simulink model "VCMGCM1962020b_v2"  (R2020b)
settings: Solver=FixedStepDiscrete  StartTime=0.0  StopTime=10.0  FixedStep=0.005  RelTol=1e-3  EnableMultiTasking=on
PreLoadFcn:
  | try, model_open; catch, disp('Error occurred while executing model pre-load callback: model_open.m'); disp('Please assure that the MATLAB working directory is set to the model directory before opening.'); end
InitFcn:
  | try, model_open; catch, end
undefined symbols (not defined in the file): Bridge, GCM, H, raptor_get_param_eval, raptor_get_safe_string, raptor_xcp_function
libraries: Blocks_lib x1165, Raptor_lib x665, simulink x62, VCM_lib x5
(part 5 of 23)

== system VCMGCM1962020b_v2/Fgnd/Diagnostics/Fault Statuses/Status Marquees ==
  f : TriggerPort  TriggerType=function-call  VariantControl=(inherit)  PortDimensions=1
  Display first 7 faults with the selected state1 : Subsystem  mask{group=group, notOccurred=off, suspected=off, active=off, occurred=off, failedThisDC=off, testCmpltThisDC=off, failing=on, pending=off, confirmed=off, mil=off, permanent=off, ready=off, prevConfirmed=off, failedSinceClear=off, failedLastDC=off, prevMil=off}
      mask prompts: notOccurred "Not Occurred"; failedThisDC "Failed This Drive Cycle"; testCmpltThisDC "Test Completed This Drive Cycle"; prevConfirmed "Previously Confirmed"; failedSinceClear "Failed Since Last Clear"; failedLastDC "FailedLastDriveCycle"; prevMil "Previously MIL"
      mask init:
      | %names used in Raptor
      | %OBD1:
      | %maskVarList = {'notOccurred' ; 'suspected'; 'active'; 'occurred'};
      | %OBD2:
      | maskVarList = {'notOccurred' ; 'suspected'; 'active'; 'occurred'; 'failedThisDC'; 'testCmpltThisDC'; 'failing'; 'pending'; 'confirmed'; 'mil'; 'permanent'; 'ready'; 'prevConfirmed'; 'failedSinceClear'; 'failedLastDC'; 'prevMil'};
      | %cleaner names to use in actual variable names
      | %OBD1:
      | %outputNameList= {'NotOccurred'; 'Suspected'; 'Active'; 'Occurred'};
      | %OBD2:
      | outputNameList = {'notOccurred' ; 'suspected'; 'active'; 'occurred'; 'FailThisDrv' ; 'CmpltThisDrv'   ; 'Failing'; 'Pending'; 'Confirmed'; 'MIL'; 'Permanent'; 'Ready'; 'PrevConfirmed'; 'FaildSinceClr'   ; 'FaildLastDrv'; 'PrevMIL'};
      | 
      | debug = [];
      | isSelected = cell(0);
      | selectedOutputNames = [];
      | for i = 1:length(maskVarList)
      |     paramVal = eval(maskVarList{i});
      |     if paramVal %if that fault is selected
      |         selectedOutputNames = [selectedOutputNames outputNameList{i}];
      |         isSelected = [isSelected 'on'];
      |     else
      |         isSelected = [isSelected 'off'];
      |     end
      | end
      | 
      | finalVarName = selectedOutputNames; %concatenate all names
      | debug = finalVarName;
      | 
      | iterators = find_system(gcb,'LookUnderMasks','all','FunctionName','raptor_sfun_fault_stateIterator');
      | countBlk = find_system(gcb,'LookUnderMasks','all','FunctionName','raptor_sfun_fault_stateCount');
      | blocks = [iterators; countBlk]; %blocks that need to be configured
      | 
      | for b = 1:length(blocks)
      |     for v = 1:length(maskVarList)
      |         set_param(blocks{b},maskVarList{v},isSelected{v});
      |     end    
      | end
      mask Display: disp(finalVarName)
  Display first 7 faults with the selected state2 : Subsystem  mask{group=group, notOccurred=off, suspected=off, active=off, occurred=off, failedThisDC=on, testCmpltThisDC=off, failing=off, pending=off, confirmed=off, mil=off, permanent=off, ready=off, prevConfirmed=off, failedSinceClear=off, failedLastDC=off, prevMil=off}
      mask prompts: notOccurred "Not Occurred"; failedThisDC "Failed This Drive Cycle"; testCmpltThisDC "Test Completed This Drive Cycle"; prevConfirmed "Previously Confirmed"; failedSinceClear "Failed Since Last Clear"; failedLastDC "FailedLastDriveCycle"; prevMil "Previously MIL"
      mask init: same as VCMGCM1962020b_v2/Fgnd/Diagnostics/Fault Statuses/Status Marquees/Display first 7 faults with the selected state1
      mask Display: disp(finalVarName)
  Fault Fail Time : Subsystem  TreatAsAtomicUnit=on
  Header : Blocks_lib/Header  width=Portrait  addtext=''
  Unit Delay{,1..6} (7 alike) : UnitDelay  SampleTime=-1  HasFrameUpgradeWarning=on
  raptor_fault_data_read : Raptor_lib/Faults/raptor_fault_data_read  dataSource=Parameter  dataName='FaultFailTime'  faultSource=Port  faultName='myFaultName'
      settings: SourceProductName=Raptor
  raptor_fault_measurement : Raptor_lib/Faults/raptor_fault_measurement  dataName='TestCompletedThisDriveCycleFaults'  calHelp='Marquee of test completed this drive cycle faults'  calAccess=1  calFunction=group
      settings: SourceProductName=Raptor
  raptor_fault_measurement1 : Raptor_lib/Faults/raptor_fault_measurement  dataName='FailingFaults'  calHelp='Marquee of failing faults'  calAccess=1  calFunction=group
      settings: SourceProductName=Raptor
  raptor_fault_measurement2 : Raptor_lib/Faults/raptor_fault_measurement  dataName='FailedThisDriveCycleFaults'  calHelp='Marquee of failed this drive cycle faults'  calAccess=1  calFunction=group
      settings: SourceProductName=Raptor
  raptor_fault_measurement3 : Raptor_lib/Faults/raptor_fault_measurement  dataName='FailedSinceClearFaults'  calHelp='Marquee of failed since clear faults'  calAccess=1  calFunction=group
      settings: SourceProductName=Raptor
  raptor_fault_measurement4 : Raptor_lib/Faults/raptor_fault_measurement  dataName='PendingFaults'  calHelp='Marquee of pending faults'  calAccess=1  calFunction=group
      settings: SourceProductName=Raptor
  raptor_fault_measurement5 : Raptor_lib/Faults/raptor_fault_measurement  dataName='ConfirmedFaults'  calHelp='Marquee of confirmed faults'  calAccess=1  calFunction=group
      settings: SourceProductName=Raptor
  raptor_fault_measurement6 : Raptor_lib/Faults/raptor_fault_measurement  dataName='PreviouslyConfirmedFaults'  calHelp='Marquee of previously confirmed faults'  calAccess=1  calFunction=group
      settings: SourceProductName=Raptor
  raptor_fault_stateIterator : Raptor_lib/Faults/raptor_fault_stateIterator  notOccurred=off  suspected=off  active=on  occurred=off  failedThisDC=off  testCmpltThisDC=on  failing=off  pending=off  confirmed=off  mil=off  permanent=off  ready=off  prevConfirmed=off  failedSinceClear=off  failedLastDC=off  prevMil=off
      settings: SourceProductName=Raptor
  raptor_fault_stateIterator1 : Raptor_lib/Faults/raptor_fault_stateIterator  notOccurred=off  suspected=off  active=on  occurred=off  failedThisDC=off  testCmpltThisDC=off  failing=on  pending=off  confirmed=off  mil=off  permanent=off  ready=off  prevConfirmed=off  failedSinceClear=off  failedLastDC=off  prevMil=off
      settings: SourceProductName=Raptor
  raptor_fault_stateIterator2 : Raptor_lib/Faults/raptor_fault_stateIterator  notOccurred=off  suspected=off  active=on  occurred=off  failedThisDC=on  testCmpltThisDC=off  failing=off  pending=off  confirmed=off  mil=off  permanent=off  ready=off  prevConfirmed=off  failedSinceClear=off  failedLastDC=off  prevMil=off
      settings: SourceProductName=Raptor
  raptor_fault_stateIterator3 : Raptor_lib/Faults/raptor_fault_stateIterator  notOccurred=off  suspected=off  active=on  occurred=off  failedThisDC=off  testCmpltThisDC=off  failing=off  pending=off  confirmed=off  mil=off  permanent=off  ready=off  prevConfirmed=off  failedSinceClear=on  failedLastDC=off  prevMil=off
      settings: SourceProductName=Raptor
  raptor_fault_stateIterator4 : Raptor_lib/Faults/raptor_fault_stateIterator  notOccurred=off  suspected=off  active=on  occurred=off  failedThisDC=off  testCmpltThisDC=off  failing=off  pending=on  confirmed=off  mil=off  permanent=off  ready=off  prevConfirmed=off  failedSinceClear=off  failedLastDC=off  prevMil=off
      settings: SourceProductName=Raptor
  raptor_fault_stateIterator5 : Raptor_lib/Faults/raptor_fault_stateIterator  notOccurred=off  suspected=off  active=on  occurred=off  failedThisDC=off  testCmpltThisDC=off  failing=off  pending=off  confirmed=on  mil=off  permanent=off  ready=off  prevConfirmed=off  failedSinceClear=off  failedLastDC=off  prevMil=off
      settings: SourceProductName=Raptor
  raptor_fault_stateIterator6 : Raptor_lib/Faults/raptor_fault_stateIterator  notOccurred=off  suspected=off  active=on  occurred=off  failedThisDC=off  testCmpltThisDC=off  failing=off  pending=off  confirmed=off  mil=off  permanent=off  ready=off  prevConfirmed=on  failedSinceClear=off  failedLastDC=off  prevMil=off
      settings: SourceProductName=Raptor
  raptor_fault_trigger : Raptor_lib/Faults/raptor_fault_trigger  triggerName='FailingTime'  setGlobal=on  stdState=Suspected  obdState=Failing  edge=Rising  alwaysEnabled=on
      settings: SourceProductName=Raptor
  raptor_measurement : Raptor_lib/Data Storage/raptor_measurement  paramName='FailedThisDriveCycleFaultsTime'  nameSource=Parameter  calDispType=Number  calEnum={'False', 'True'}  calGain=1.0  calOffset=0.0  calMax=inf  calMin=-inf  calFormat='-1'  calUnit='Marquee of failed this drive cycle faults time'  calHelp='sec'  calAccess=1  calFunction=group  calVisible=on
      settings: SourceProductName=Raptor
  wires:
  raptor_fault_stateIterator/1 -> raptor_fault_measurement/1, Unit Delay/1
  Unit Delay/1 -> raptor_fault_stateIterator/1
  Unit Delay1/1 -> raptor_fault_stateIterator1/1
  raptor_fault_stateIterator1/1 -> Unit Delay1/1, raptor_fault_measurement1/1
  raptor_fault_stateIterator2/1 -> raptor_fault_measurement2/1, raptor_fault_data_read/1, Unit Delay2/1
  Unit Delay2/1 -> raptor_fault_stateIterator2/1
  Unit Delay3/1 -> raptor_fault_stateIterator3/1
  raptor_fault_stateIterator3/1 -> Unit Delay3/1, raptor_fault_measurement3/1
  raptor_fault_stateIterator4/1 -> raptor_fault_measurement4/1, Unit Delay4/1
  Unit Delay4/1 -> raptor_fault_stateIterator4/1
  Unit Delay5/1 -> raptor_fault_stateIterator5/1
  raptor_fault_stateIterator5/1 -> Unit Delay5/1, raptor_fault_measurement5/1
  raptor_fault_stateIterator6/1 -> raptor_fault_measurement6/1, Unit Delay6/1
  Unit Delay6/1 -> raptor_fault_stateIterator6/1
  raptor_fault_trigger/2 -> Fault Fail Time/1(Idx)
  raptor_fault_trigger/1 -> Fault Fail Time/Trigger
  raptor_fault_data_read/1 -> raptor_measurement/1

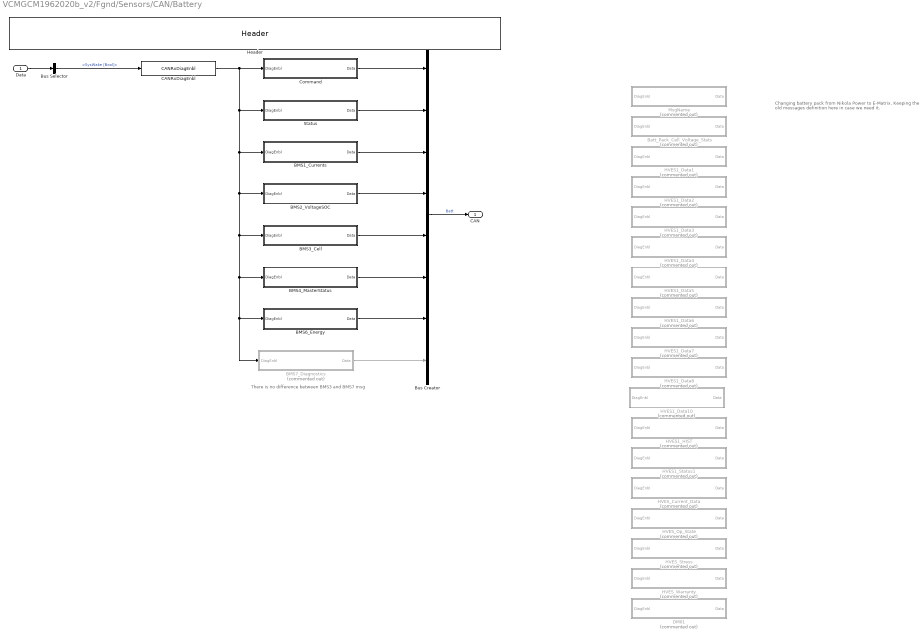
== system VCMGCM1962020b_v2/Fgnd/Sensors/CAN/Battery ==
  note: There is no difference between BMS3 and BMS7 msg
  note: Changing battery pack from Nikola Power to E-Matrix.
      | Keeping the old messages definition here in case we need it.
  Data : Inport
  BMS1_Currents : Subsystem  mask{samptime=samptime}
      mask prompts: samptime "Sample Time (sec)"
      mask help:
      | Example of how to set up a CAN message recieve.
      | 1. Copy this block into the main model.
      | 2. Disable/break library link.
      | 3. Underneath, set up CAN Rx Message block.
      | 4. For each field, connect a CANRxField block from the CAN block to the bus creator; adjust parameters as necessary.
      mask init:
      | [msgnam, msgbus] = CANBlockInit('Rx');
      mask Display: disp(['CAN Rx: Message\n' msgnam '\n' msgbus]);
  BMS2_VoltageSOC : Subsystem  AncestorBlock=Blocks_lib/MsgName5  mask{samptime=0.005}
      mask prompts: samptime "Sample Time (sec)"
      mask help:
      | Example of how to set up a CAN message recieve.
      | 1. Copy this block into the main model.
      | 2. Disable/break library link.
      | 3. Underneath, set up CAN Rx Message block.
      | 4. For each field, connect a CANRxField block from the CAN block to the bus creator; adjust parameters as necessary.
      mask init:
      | [msgnam, msgbus] = CANBlockInit('Rx');
      mask Display: disp(['CAN Rx: Message\n' msgnam '\n' msgbus]);
  BMS3_Cell : Subsystem  mask{samptime=samptime}
      mask prompts: samptime "Sample Time (sec)"
      mask help:
      | Example of how to set up a CAN message recieve.
      | 1. Copy this block into the main model.
      | 2. Disable/break library link.
      | 3. Underneath, set up CAN Rx Message block.
      | 4. For each field, connect a CANRxField block from the CAN block to the bus creator; adjust parameters as necessary.
      mask init:
      | [msgnam, msgbus] = CANBlockInit('Rx');
      mask Display: disp(['CAN Rx: Message\n' msgnam '\n' msgbus]);
  BMS4_MasterStatus : Subsystem  mask{samptime=samptime}
      mask prompts: samptime "Sample Time (sec)"
      mask help:
      | Example of how to set up a CAN message recieve.
      | 1. Copy this block into the main model.
      | 2. Disable/break library link.
      | 3. Underneath, set up CAN Rx Message block.
      | 4. For each field, connect a CANRxField block from the CAN block to the bus creator; adjust parameters as necessary.
      mask init:
      | [msgnam, msgbus] = CANBlockInit('Rx');
      mask Display: disp(['CAN Rx: Message\n' msgnam '\n' msgbus]);
  BMS6_Energy : Subsystem  mask{samptime=samptime}
      mask prompts: samptime "Sample Time (sec)"
      mask help:
      | Example of how to set up a CAN message recieve.
      | 1. Copy this block into the main model.
      | 2. Disable/break library link.
      | 3. Underneath, set up CAN Rx Message block.
      | 4. For each field, connect a CANRxField block from the CAN block to the bus creator; adjust parameters as necessary.
      mask init:
      | [msgnam, msgbus] = CANBlockInit('Rx');
      mask Display: disp(['CAN Rx: Message\n' msgnam '\n' msgbus]);
  BMS7_Diagnostics : Subsystem  Commented=on  mask{samptime=samptime}
      mask prompts: samptime "Sample Time (sec)"
      mask help:
      | Example of how to set up a CAN message recieve.
      | 1. Copy this block into the main model.
      | 2. Disable/break library link.
      | 3. Underneath, set up CAN Rx Message block.
      | 4. For each field, connect a CANRxField block from the CAN block to the bus creator; adjust parameters as necessary.
      mask init:
      | [msgnam, msgbus] = CANBlockInit('Rx');
      mask Display: disp(['CAN Rx: Message\n' msgnam '\n' msgbus]);
  Batt_Pack_Cell_Voltage_Stats : Subsystem  Commented=on  mask{samptime=samptime}
      mask prompts: samptime "Sample Time (sec)"
      mask help:
      | Example of how to set up a CAN message recieve.
      | 1. Copy this block into the main model.
      | 2. Disable/break library link.
      | 3. Underneath, set up CAN Rx Message block.
      | 4. For each field, connect a CANRxField block from the CAN block to the bus creator; adjust parameters as necessary.
      mask init:
      | [msgnam, msgbus] = CANBlockInit('Rx');
      mask Display: disp(['CAN Rx: Message\n' msgnam '\n' msgbus]);
  Bus Creator : BusCreator  Inputs=8
  Bus Selector : BusSelector  OutputSignals=Control.Other.Other.SysWake [Bool]
  CANRxDiagEnbl : Blocks_lib/CANRxDiagEnbl  nam='Batt'
  Command : Subsystem  mask{samptime=samptime}
      mask prompts: samptime "Sample Time (sec)"
      mask help:
      | Example of how to set up a CAN message recieve.
      | 1. Copy this block into the main model.
      | 2. Disable/break library link.
      | 3. Underneath, set up CAN Rx Message block.
      | 4. For each field, connect a CANRxField block from the CAN block to the bus creator; adjust parameters as necessary.
      mask init:
      | [msgnam, msgbus] = CANBlockInit('Rx');
      mask Display: disp(['CAN Rx: Message\n' msgnam '\n' msgbus]);
  DM01 : Subsystem  Commented=on  mask{samptime=samptime}
      mask prompts: samptime "Sample Time (sec)"
      mask help:
      | Example of how to set up a CAN message recieve.
      | 1. Copy this block into the main model.
      | 2. Disable/break library link.
      | 3. Underneath, set up CAN Rx Message block.
      | 4. For each field, connect a CANRxField block from the CAN block to the bus creator; adjust parameters as necessary.
      mask init:
      | [msgnam, msgbus] = CANBlockInit('Rx');
      mask Display: disp(['CAN Rx: Message\n' msgnam '\n' msgbus]);
  HVES1_Data1 : Subsystem  Commented=on  mask{samptime=samptime}
      mask prompts: samptime "Sample Time (sec)"
      mask help:
      | Example of how to set up a CAN message recieve.
      | 1. Copy this block into the main model.
      | 2. Disable/break library link.
      | 3. Underneath, set up CAN Rx Message block.
      | 4. For each field, connect a CANRxField block from the CAN block to the bus creator; adjust parameters as necessary.
      mask init:
      | [msgnam, msgbus] = CANBlockInit('Rx');
      mask Display: disp(['CAN Rx: Message\n' msgnam '\n' msgbus]);
  HVES1_Data10 : Subsystem  Commented=on  mask{samptime=samptime}
      mask prompts: samptime "Sample Time (sec)"
      mask help:
      | Example of how to set up a CAN message recieve.
      | 1. Copy this block into the main model.
      | 2. Disable/break library link.
      | 3. Underneath, set up CAN Rx Message block.
      | 4. For each field, connect a CANRxField block from the CAN block to the bus creator; adjust parameters as necessary.
      mask init:
      | [msgnam, msgbus] = CANBlockInit('Rx');
      mask Display: disp(['CAN Rx: Message\n' msgnam '\n' msgbus]);
  HVES1_Data2 : Subsystem  Commented=on  mask{samptime=samptime}
      mask prompts: samptime "Sample Time (sec)"
      mask help:
      | Example of how to set up a CAN message recieve.
      | 1. Copy this block into the main model.
      | 2. Disable/break library link.
      | 3. Underneath, set up CAN Rx Message block.
      | 4. For each field, connect a CANRxField block from the CAN block to the bus creator; adjust parameters as necessary.
      mask init:
      | [msgnam, msgbus] = CANBlockInit('Rx');
      mask Display: disp(['CAN Rx: Message\n' msgnam '\n' msgbus]);
  HVES1_Data3 : Subsystem  Commented=on  mask{samptime=samptime}
      mask prompts: samptime "Sample Time (sec)"
      mask help:
      | Example of how to set up a CAN message recieve.
      | 1. Copy this block into the main model.
      | 2. Disable/break library link.
      | 3. Underneath, set up CAN Rx Message block.
      | 4. For each field, connect a CANRxField block from the CAN block to the bus creator; adjust parameters as necessary.
      mask init:
      | [msgnam, msgbus] = CANBlockInit('Rx');
      mask Display: disp(['CAN Rx: Message\n' msgnam '\n' msgbus]);
  HVES1_Data4 : Subsystem  Commented=on  mask{samptime=samptime}
      mask prompts: samptime "Sample Time (sec)"
      mask help:
      | Example of how to set up a CAN message recieve.
      | 1. Copy this block into the main model.
      | 2. Disable/break library link.
      | 3. Underneath, set up CAN Rx Message block.
      | 4. For each field, connect a CANRxField block from the CAN block to the bus creator; adjust parameters as necessary.
      mask init:
      | [msgnam, msgbus] = CANBlockInit('Rx');
      mask Display: disp(['CAN Rx: Message\n' msgnam '\n' msgbus]);
  HVES1_Data5 : Subsystem  Commented=on  mask{samptime=samptime}
      mask prompts: samptime "Sample Time (sec)"
      mask help:
      | Example of how to set up a CAN message recieve.
      | 1. Copy this block into the main model.
      | 2. Disable/break library link.
      | 3. Underneath, set up CAN Rx Message block.
      | 4. For each field, connect a CANRxField block from the CAN block to the bus creator; adjust parameters as necessary.
      mask init:
      | [msgnam, msgbus] = CANBlockInit('Rx');
      mask Display: disp(['CAN Rx: Message\n' msgnam '\n' msgbus]);
  HVES1_Data6 : Subsystem  Commented=on  mask{samptime=samptime}
      mask prompts: samptime "Sample Time (sec)"
      mask help:
      | Example of how to set up a CAN message recieve.
      | 1. Copy this block into the main model.
      | 2. Disable/break library link.
      | 3. Underneath, set up CAN Rx Message block.
      | 4. For each field, connect a CANRxField block from the CAN block to the bus creator; adjust parameters as necessary.
      mask init:
      | [msgnam, msgbus] = CANBlockInit('Rx');
      mask Display: disp(['CAN Rx: Message\n' msgnam '\n' msgbus]);
  HVES1_Data7 : Subsystem  Commented=on  mask{samptime=samptime}
      mask prompts: samptime "Sample Time (sec)"
      mask help:
      | Example of how to set up a CAN message recieve.
      | 1. Copy this block into the main model.
      | 2. Disable/break library link.
      | 3. Underneath, set up CAN Rx Message block.
      | 4. For each field, connect a CANRxField block from the CAN block to the bus creator; adjust parameters as necessary.
      mask init:
      | [msgnam, msgbus] = CANBlockInit('Rx');
      mask Display: disp(['CAN Rx: Message\n' msgnam '\n' msgbus]);
  HVES1_Data8 : Subsystem  Commented=on  mask{samptime=samptime}
      mask prompts: samptime "Sample Time (sec)"
      mask help:
      | Example of how to set up a CAN message recieve.
      | 1. Copy this block into the main model.
      | 2. Disable/break library link.
      | 3. Underneath, set up CAN Rx Message block.
      | 4. For each field, connect a CANRxField block from the CAN block to the bus creator; adjust parameters as necessary.
      mask init:
      | [msgnam, msgbus] = CANBlockInit('Rx');
      mask Display: disp(['CAN Rx: Message\n' msgnam '\n' msgbus]);
  HVES1_HIST : Subsystem  Commented=on  mask{samptime=samptime}
      mask prompts: samptime "Sample Time (sec)"
      mask help:
      | Example of how to set up a CAN message recieve.
      | 1. Copy this block into the main model.
      | 2. Disable/break library link.
      | 3. Underneath, set up CAN Rx Message block.
      | 4. For each field, connect a CANRxField block from the CAN block to the bus creator; adjust parameters as necessary.
      mask init:
      | [msgnam, msgbus] = CANBlockInit('Rx');
      mask Display: disp(['CAN Rx: Message\n' msgnam '\n' msgbus]);
  HVES1_Status1 : Subsystem  Commented=on  mask{samptime=samptime}
      mask prompts: samptime "Sample Time (sec)"
      mask help:
      | Example of how to set up a CAN message recieve.
      | 1. Copy this block into the main model.
      | 2. Disable/break library link.
      | 3. Underneath, set up CAN Rx Message block.
      | 4. For each field, connect a CANRxField block from the CAN block to the bus creator; adjust parameters as necessary.
      mask init:
      | [msgnam, msgbus] = CANBlockInit('Rx');
      mask Display: disp(['CAN Rx: Message\n' msgnam '\n' msgbus]);
  HVES_Current_Data : Subsystem  Commented=on  mask{samptime=samptime}
      mask prompts: samptime "Sample Time (sec)"
      mask help:
      | Example of how to set up a CAN message recieve.
      | 1. Copy this block into the main model.
      | 2. Disable/break library link.
      | 3. Underneath, set up CAN Rx Message block.
      | 4. For each field, connect a CANRxField block from the CAN block to the bus creator; adjust parameters as necessary.
      mask init:
      | [msgnam, msgbus] = CANBlockInit('Rx');
      mask Display: disp(['CAN Rx: Message\n' msgnam '\n' msgbus]);
  HVES_Op_State : Subsystem  Commented=on  mask{samptime=samptime}
      mask prompts: samptime "Sample Time (sec)"
      mask help:
      | Example of how to set up a CAN message recieve.
      | 1. Copy this block into the main model.
      | 2. Disable/break library link.
      | 3. Underneath, set up CAN Rx Message block.
      | 4. For each field, connect a CANRxField block from the CAN block to the bus creator; adjust parameters as necessary.
      mask init:
      | [msgnam, msgbus] = CANBlockInit('Rx');
      mask Display: disp(['CAN Rx: Message\n' msgnam '\n' msgbus]);
  HVES_Stress : Subsystem  Commented=on  mask{samptime=samptime}
      mask prompts: samptime "Sample Time (sec)"
      mask help:
      | Example of how to set up a CAN message recieve.
      | 1. Copy this block into the main model.
      | 2. Disable/break library link.
      | 3. Underneath, set up CAN Rx Message block.
      | 4. For each field, connect a CANRxField block from the CAN block to the bus creator; adjust parameters as necessary.
      mask init:
      | [msgnam, msgbus] = CANBlockInit('Rx');
      mask Display: disp(['CAN Rx: Message\n' msgnam '\n' msgbus]);
  HVES_Warranty : Subsystem  Commented=on  mask{samptime=samptime}
      mask prompts: samptime "Sample Time (sec)"
      mask help:
      | Example of how to set up a CAN message recieve.
      | 1. Copy this block into the main model.
      | 2. Disable/break library link.
      | 3. Underneath, set up CAN Rx Message block.
      | 4. For each field, connect a CANRxField block from the CAN block to the bus creator; adjust parameters as necessary.
      mask init:
      | [msgnam, msgbus] = CANBlockInit('Rx');
      mask Display: disp(['CAN Rx: Message\n' msgnam '\n' msgbus]);
  Header : Blocks_lib/Header  width=Portrait  addtext=''
  MsgName : Subsystem  Commented=on  mask{samptime=samptime}
      mask prompts: samptime "Sample Time (sec)"
      mask help:
      | Example of how to set up a CAN message recieve.
      | 1. Copy this block into the main model.
      | 2. Disable/break library link.
      | 3. Underneath, set up CAN Rx Message block.
      | 4. For each field, connect a CANRxField block from the CAN block to the bus creator; adjust parameters as necessary.
      mask init:
      | [msgnam, msgbus] = CANBlockInit('Rx');
      mask Display: disp(['CAN Rx: Message\n' msgnam '\n' msgbus]);
  Status : Subsystem  mask{samptime=samptime}
      mask prompts: samptime "Sample Time (sec)"
      mask help:
      | Example of how to set up a CAN message recieve.
      | 1. Copy this block into the main model.
      | 2. Disable/break library link.
      | 3. Underneath, set up CAN Rx Message block.
      | 4. For each field, connect a CANRxField block from the CAN block to the bus creator; adjust parameters as necessary.
      mask init:
      | [msgnam, msgbus] = CANBlockInit('Rx');
      mask Display: disp(['CAN Rx: Message\n' msgnam '\n' msgbus]);
  CAN : Outport  VectorParamsAs1DForOutWhenUnconnected=off
  wires:
  Bus Creator/1 -> CAN/1  "Batt"
  Bus Selector/1 -> CANRxDiagEnbl/1  "<SysWake [Bool]>"
  Data/1 -> Bus Selector/1
  BMS3_Cell/1(Data) -> Bus Creator/5
  CANRxDiagEnbl/1 -> Command/1(DiagEnbl), BMS1_Currents/1(DiagEnbl), BMS2_VoltageSOC/1(DiagEnbl), BMS7_Diagnostics/1(DiagEnbl), BMS6_Energy/1(DiagEnbl), BMS4_MasterStatus/1(DiagEnbl), BMS3_Cell/1(DiagEnbl), Status/1(DiagEnbl)
  Command/1(Data) -> Bus Creator/1
  BMS2_VoltageSOC/1(Data) -> Bus Creator/4
  Status/1(Data) -> Bus Creator/2
  BMS4_MasterStatus/1(Data) -> Bus Creator/6
  BMS6_Energy/1(Data) -> Bus Creator/7
  BMS7_Diagnostics/1(Data) -> Bus Creator/8
  BMS1_Currents/1(Data) -> Bus Creator/3

== system VCMGCM1962020b_v2/Fgnd/Sensors/CAN/CCS Interface ==
  Data : Inport
  Bus Creator : BusCreator  Inputs=8
  Bus Selector : BusSelector  OutputSignals=Control.Mode.StartStop.ChgCycle [Bool],Control.Mode.StartStop.ModWake [Bool]
  CANRxDiagEnbl : Blocks_lib/CANRxDiagEnbl  nam=nam
  CCSEVSE_ChargeParameters1 : Subsystem  mask{samptime=samptime}
      mask prompts: samptime "Sample Time (sec)"
      mask help:
      | Example of how to set up a CAN message recieve.
      | 1. Copy this block into the main model.
      | 2. Disable/break library link.
      | 3. Underneath, set up CAN Rx Message block.
      | 4. For each field, connect a CANRxField block from the CAN block to the bus creator; adjust parameters as necessary.
      mask init:
      | [msgnam, msgbus] = CANBlockInit('Rx');
      mask Display: disp(['CAN Rx: Message\n' msgnam '\n' msgbus]);
  CCSEVSE_ChargeParameters2 : Subsystem  mask{samptime=samptime}
      mask prompts: samptime "Sample Time (sec)"
      mask help:
      | Example of how to set up a CAN message recieve.
      | 1. Copy this block into the main model.
      | 2. Disable/break library link.
      | 3. Underneath, set up CAN Rx Message block.
      | 4. For each field, connect a CANRxField block from the CAN block to the bus creator; adjust parameters as necessary.
      mask init:
      | [msgnam, msgbus] = CANBlockInit('Rx');
      mask Display: disp(['CAN Rx: Message\n' msgnam '\n' msgbus]);
  CCSEVSE_DC_ChargeInfo1 : Subsystem  mask{samptime=samptime}
      mask prompts: samptime "Sample Time (sec)"
      mask help:
      | Example of how to set up a CAN message recieve.
      | 1. Copy this block into the main model.
      | 2. Disable/break library link.
      | 3. Underneath, set up CAN Rx Message block.
      | 4. For each field, connect a CANRxField block from the CAN block to the bus creator; adjust parameters as necessary.
      mask init:
      | [msgnam, msgbus] = CANBlockInit('Rx');
      mask Display: disp(['CAN Rx: Message\n' msgnam '\n' msgbus]);
  CCSM2IEV_Alerts : Subsystem  mask{samptime=samptime}
      mask prompts: samptime "Sample Time (sec)"
      mask help:
      | Example of how to set up a CAN message recieve.
      | 1. Copy this block into the main model.
      | 2. Disable/break library link.
      | 3. Underneath, set up CAN Rx Message block.
      | 4. For each field, connect a CANRxField block from the CAN block to the bus creator; adjust parameters as necessary.
      mask init:
      | [msgnam, msgbus] = CANBlockInit('Rx');
      mask Display: disp(['CAN Rx: Message\n' msgnam '\n' msgbus]);
  CCSM2IEV_Command : Subsystem  mask{samptime=samptime}
      mask prompts: samptime "Sample Time (sec)"
      mask help:
      | Example of how to set up a CAN message recieve.
      | 1. Copy this block into the main model.
      | 2. Disable/break library link.
      | 3. Underneath, set up CAN Rx Message block.
      | 4. For each field, connect a CANRxField block from the CAN block to the bus creator; adjust parameters as necessary.
      mask init:
      | [msgnam, msgbus] = CANBlockInit('Rx');
      mask Display: disp(['CAN Rx: Message\n' msgnam '\n' msgbus]);
  CCSM2IEV_Info : Subsystem  mask{samptime=samptime}
      mask prompts: samptime "Sample Time (sec)"
      mask help:
      | Example of how to set up a CAN message recieve.
      | 1. Copy this block into the main model.
      | 2. Disable/break library link.
      | 3. Underneath, set up CAN Rx Message block.
      | 4. For each field, connect a CANRxField block from the CAN block to the bus creator; adjust parameters as necessary.
      mask init:
      | [msgnam, msgbus] = CANBlockInit('Rx');
      mask Display: disp(['CAN Rx: Message\n' msgnam '\n' msgbus]);
  CCSM2IEV_TemperatureInfo : Subsystem  mask{samptime=samptime}
      mask prompts: samptime "Sample Time (sec)"
      mask help:
      | Example of how to set up a CAN message recieve.
      | 1. Copy this block into the main model.
      | 2. Disable/break library link.
      | 3. Underneath, set up CAN Rx Message block.
      | 4. For each field, connect a CANRxField block from the CAN block to the bus creator; adjust parameters as necessary.
      mask init:
      | [msgnam, msgbus] = CANBlockInit('Rx');
      mask Display: disp(['CAN Rx: Message\n' msgnam '\n' msgbus]);
  Header : Blocks_lib/Header  width=Portrait  addtext=''
  Logical Operator : Logic  AllPortsSameDT=off  OutDataTypeStr=boolean
  MsgName : Subsystem  mask{samptime=samptime}
      mask prompts: samptime "Sample Time (sec)"
      mask help:
      | Example of how to set up a CAN message recieve.
      | 1. Copy this block into the main model.
      | 2. Disable/break library link.
      | 3. Underneath, set up CAN Rx Message block.
      | 4. For each field, connect a CANRxField block from the CAN block to the bus creator; adjust parameters as necessary.
      mask init:
      | [msgnam, msgbus] = CANBlockInit('Rx');
      mask Display: disp(['CAN Rx: Message\n' msgnam '\n' msgbus]);
  CAN : Outport  VectorParamsAs1DForOutWhenUnconnected=off
  wires:
  CCSEVSE_ChargeParameters1/1(Data) -> Bus Creator/6
  CCSM2IEV_TemperatureInfo/1(Data) -> Bus Creator/8
  CCSEVSE_ChargeParameters2/1(Data) -> Bus Creator/7
  MsgName/1(Data) -> Bus Creator/5
  CCSEVSE_DC_ChargeInfo1/1(Data) -> Bus Creator/4
  CCSM2IEV_Alerts/1(Data) -> Bus Creator/3
  CCSM2IEV_Command/1(Data) -> Bus Creator/2
  CCSM2IEV_Info/1(Data) -> Bus Creator/1
  Data/1 -> Bus Selector/1
  Bus Creator/1 -> CAN/1  "CCS"
  CANRxDiagEnbl/1 -> CCSM2IEV_Info/1(DiagEnbl), CCSM2IEV_Command/1(DiagEnbl), CCSM2IEV_Alerts/1(DiagEnbl), CCSEVSE_DC_ChargeInfo1/1(DiagEnbl), MsgName/1(DiagEnbl), CCSEVSE_ChargeParameters1/1(DiagEnbl), CCSEVSE_ChargeParameters2/1(DiagEnbl), CCSM2IEV_TemperatureInfo/1(DiagEnbl)
  Bus Selector/1 -> Logical Operator/1  "<ChgCycle [Bool]>"
  Bus Selector/2 -> Logical Operator/2  "<ModWake [Bool]>"
  Logical Operator/1 -> CANRxDiagEnbl/1

== system VCMGCM1962020b_v2/Fgnd/Sensors/CAN/Charger ==
  Data : Inport
  Bus Creator : BusCreator  Inputs=3
  Bus Selector : BusSelector  OutputSignals=Sensors.Sensors.Volt.WakeChgr.WakeChgr [Bool],VirtualSensors.Chgr.OnBoard.OnBoardChgr [Bool]
  CANRxDiagEnbl : Blocks_lib/CANRxDiagEnbl  nam=nam
  ChgrCCSA : Subsystem  mask{samptime=samptime}
      mask prompts: samptime "Sample Time (sec)"
      mask help:
      | Example of how to set up a CAN message recieve.
      | 1. Copy this block into the main model.
      | 2. Disable/break library link.
      | 3. Underneath, set up CAN Rx Message block.
      | 4. For each field, connect a CANRxField block from the CAN block to the bus creator; adjust parameters as necessary.
      mask init:
      | [msgnam, msgbus] = CANBlockInit('Rx');
      mask Display: disp(['CAN Rx: Message\n' msgnam '\n' msgbus]);
  ChgrCCSB : Subsystem  mask{samptime=samptime}
      mask prompts: samptime "Sample Time (sec)"
      mask help:
      | Example of how to set up a CAN message recieve.
      | 1. Copy this block into the main model.
      | 2. Disable/break library link.
      | 3. Underneath, set up CAN Rx Message block.
      | 4. For each field, connect a CANRxField block from the CAN block to the bus creator; adjust parameters as necessary.
      mask init:
      | [msgnam, msgbus] = CANBlockInit('Rx');
      mask Display: disp(['CAN Rx: Message\n' msgnam '\n' msgbus]);
  ChgrCCSC : Subsystem  mask{samptime=samptime}
      mask prompts: samptime "Sample Time (sec)"
      mask help:
      | Example of how to set up a CAN message recieve.
      | 1. Copy this block into the main model.
      | 2. Disable/break library link.
      | 3. Underneath, set up CAN Rx Message block.
      | 4. For each field, connect a CANRxField block from the CAN block to the bus creator; adjust parameters as necessary.
      mask init:
      | [msgnam, msgbus] = CANBlockInit('Rx');
      mask Display: disp(['CAN Rx: Message\n' msgnam '\n' msgbus]);
  Header : Blocks_lib/Header  width=Portrait  addtext=''
  Logical Operator : Logic  AllPortsSameDT=off  OutDataTypeStr=boolean
  CAN : Outport  VectorParamsAs1DForOutWhenUnconnected=off
  wires:
  Logical Operator/1 -> CANRxDiagEnbl/1
  Bus Selector/2 -> Logical Operator/2  "<OnBoardChgr [Bool]>"
  Bus Selector/1 -> Logical Operator/1  "<WakeChgr [Bool]>"
  Data/1 -> Bus Selector/1
  ChgrCCSB/1(Data) -> Bus Creator/2
  ChgrCCSA/1(Data) -> Bus Creator/1
  Bus Creator/1 -> CAN/1  "OnBoardChgr"
  CANRxDiagEnbl/1 -> ChgrCCSA/1(DiagEnbl), ChgrCCSC/1(DiagEnbl), ChgrCCSB/1(DiagEnbl)
  ChgrCCSC/1(Data) -> Bus Creator/3

== system VCMGCM1962020b_v2/Fgnd/Sensors/CAN/DC//DC Converter ==
  Data : Inport
  Bus Creator : BusCreator  Inputs=1
  Bus Selector : BusSelector  OutputSignals=Control.Other.Other.SysWake [Bool]
  CANRxDiagEnbl : Blocks_lib/CANRxDiagEnbl  nam=nam
  DCDC_Status_0_16V : Subsystem  mask{samptime=samptime}
      mask prompts: samptime "Sample Time (sec)"
      mask help:
      | Example of how to set up a CAN message recieve.
      | 1. Copy this block into the main model.
      | 2. Disable/break library link.
      | 3. Underneath, set up CAN Rx Message block.
      | 4. For each field, connect a CANRxField block from the CAN block to the bus creator; adjust parameters as necessary.
      mask init:
      | [msgnam, msgbus] = CANBlockInit('Rx');
      mask Display: disp(['CAN Rx: Message\n' msgnam '\n' msgbus]);
  Header : Blocks_lib/Header  width=Portrait  addtext=''
  CAN : Outport  VectorParamsAs1DForOutWhenUnconnected=off
  wires:
  Bus Creator/1 -> CAN/1  "DCDC"
  DCDC_Status_0_16V/1(Data) -> Bus Creator/1
  Bus Selector/1 -> CANRxDiagEnbl/1  "<SysWake [Bool]>"
  Data/1 -> Bus Selector/1
  CANRxDiagEnbl/1 -> DCDC_Status_0_16V/1(DiagEnbl)

== system VCMGCM1962020b_v2/Fgnd/Sensors/CAN/Inverter ==
  Data : Inport
  Bus Creator : BusCreator  Inputs=5
  Bus Selector : BusSelector  OutputSignals=Control.Other.Other.SysWake [Bool]
  CANRxDiagEnbl : Blocks_lib/CANRxDiagEnbl  nam='Invrtr2'
  EM1 : Subsystem  mask{samptime=samptime}
      mask prompts: samptime "Sample Time (sec)"
      mask help:
      | Example of how to set up a CAN message recieve.
      | 1. Copy this block into the main model.
      | 2. Disable/break library link.
      | 3. Underneath, set up CAN Rx Message block.
      | 4. For each field, connect a CANRxField block from the CAN block to the bus creator; adjust parameters as necessary.
      mask init:
      | [msgnam, msgbus] = CANBlockInit('Rx');
      mask Display: disp(['CAN Rx: Message\n' msgnam '\n' msgbus]);
  EM2_InvTemp : Subsystem  mask{samptime=samptime}
      mask prompts: samptime "Sample Time (sec)"
      mask help:
      | Example of how to set up a CAN message recieve.
      | 1. Copy this block into the main model.
      | 2. Disable/break library link.
      | 3. Underneath, set up CAN Rx Message block.
      | 4. For each field, connect a CANRxField block from the CAN block to the bus creator; adjust parameters as necessary.
      mask init:
      | [msgnam, msgbus] = CANBlockInit('Rx');
      mask Display: disp(['CAN Rx: Message\n' msgnam '\n' msgbus]);
  EM3 : Subsystem  Commented=on  mask{samptime=samptime}
      mask prompts: samptime "Sample Time (sec)"
      mask help:
      | Example of how to set up a CAN message recieve.
      | 1. Copy this block into the main model.
      | 2. Disable/break library link.
      | 3. Underneath, set up CAN Rx Message block.
      | 4. For each field, connect a CANRxField block from the CAN block to the bus creator; adjust parameters as necessary.
      mask init:
      | [msgnam, msgbus] = CANBlockInit('Rx');
      mask Display: disp(['CAN Rx: Message\n' msgnam '\n' msgbus]);
  EM3_DCV : Subsystem  mask{samptime=samptime}
      mask prompts: samptime "Sample Time (sec)"
      mask help:
      | Example of how to set up a CAN message recieve.
      | 1. Copy this block into the main model.
      | 2. Disable/break library link.
      | 3. Underneath, set up CAN Rx Message block.
      | 4. For each field, connect a CANRxField block from the CAN block to the bus creator; adjust parameters as necessary.
      mask init:
      | [msgnam, msgbus] = CANBlockInit('Rx');
      mask Display: disp(['CAN Rx: Message\n' msgnam '\n' msgbus]);
  EM4 : Subsystem  Commented=on  mask{samptime=samptime}
      mask prompts: samptime "Sample Time (sec)"
      mask help:
      | Example of how to set up a CAN message recieve.
      | 1. Copy this block into the main model.
      | 2. Disable/break library link.
      | 3. Underneath, set up CAN Rx Message block.
      | 4. For each field, connect a CANRxField block from the CAN block to the bus creator; adjust parameters as necessary.
      mask init:
      | [msgnam, msgbus] = CANBlockInit('Rx');
      mask Display: disp(['CAN Rx: Message\n' msgnam '\n' msgbus]);
  EM4_Spd : Subsystem  mask{samptime=samptime}
      mask prompts: samptime "Sample Time (sec)"
      mask help:
      | Example of how to set up a CAN message recieve.
      | 1. Copy this block into the main model.
      | 2. Disable/break library link.
      | 3. Underneath, set up CAN Rx Message block.
      | 4. For each field, connect a CANRxField block from the CAN block to the bus creator; adjust parameters as necessary.
      mask init:
      | [msgnam, msgbus] = CANBlockInit('Rx');
      mask Display: disp(['CAN Rx: Message\n' msgnam '\n' msgbus]);
  EM_BOOT : Subsystem  mask{samptime=samptime}
      mask prompts: samptime "Sample Time (sec)"
      mask help:
      | Example of how to set up a CAN message recieve.
      | 1. Copy this block into the main model.
      | 2. Disable/break library link.
      | 3. Underneath, set up CAN Rx Message block.
      | 4. For each field, connect a CANRxField block from the CAN block to the bus creator; adjust parameters as necessary.
      mask init:
      | [msgnam, msgbus] = CANBlockInit('Rx');
      mask Display: disp(['CAN Rx: Message\n' msgnam '\n' msgbus]);
  Header : Blocks_lib/Header  width=Portrait  addtext=''
  MsgName : Subsystem  Commented=on  mask{samptime=samptime}
      mask prompts: samptime "Sample Time (sec)"
      mask help:
      | Example of how to set up a CAN message recieve.
      | 1. Copy this block into the main model.
      | 2. Disable/break library link.
      | 3. Underneath, set up CAN Rx Message block.
      | 4. For each field, connect a CANRxField block from the CAN block to the bus creator; adjust parameters as necessary.
      mask init:
      | [msgnam, msgbus] = CANBlockInit('Rx');
      mask Display: disp(['CAN Rx: Message\n' msgnam '\n' msgbus]);
  CAN : Outport  VectorParamsAs1DForOutWhenUnconnected=off
  wires:
  EM1/1(Data) -> Bus Creator/1
  Bus Creator/1 -> CAN/1  "DrvInvtr"
  Bus Selector/1 -> CANRxDiagEnbl/1  "<SysWake [Bool]>"
  Data/1 -> Bus Selector/1
  CANRxDiagEnbl/1 -> EM2_InvTemp/1(DiagEnbl), EM4_Spd/1(DiagEnbl), EM3_DCV/1(DiagEnbl), EM_BOOT/1(DiagEnbl), EM1/1(DiagEnbl)
  EM_BOOT/1(Data) -> Bus Creator/2
  EM2_InvTemp/1(Output) -> Bus Creator/3
  EM3_DCV/1(Output) -> Bus Creator/4
  EM4_Spd/1(Output) -> Bus Creator/5

== system VCMGCM1962020b_v2/Fgnd/Sensors/CAN/Other ==
  Data : Inport
  A/C Compressor : Subsystem  Commented=on  mask{nam='ACC', bus='CAN1'}
      mask prompts: nam "Name"; bus "CAN Bus"
      mask init:
      | cb = gcb;
      | 
      | % --- Name Line
      | NameLine([cb '/CAN'], 'Inport', nam);
      mask Display: disp(['A/C Comp.: Mitsubishi EV36BNx\n' nam '\n' bus]);
  BCM : Subsystem  mask{nam='BCM', bus='CAN1'}
      mask prompts: nam "Name"; bus "CAN Bus"
      mask init:
      | cb = gcb;
      | 
      | % --- Name Line
      | NameLine([cb '/CAN'], 'Inport', nam);
      mask Display: disp(['Body Control\n' nam '\n' bus]);
  BCM1 : Subsystem  mask{nam='Display', bus='CAN1'}
      mask prompts: nam "Name"; bus "CAN Bus"
      mask init:
      | cb = gcb;
      | 
      | % --- Name Line
      | NameLine([cb '/CAN'], 'Inport', nam);
      mask Display: disp(['Display\n' nam '\n' bus]);
  Bus Creator : BusCreator  Inputs=4
  Charge Port DC Voltage Sensor : Subsystem  mask{bus='CAN1'}
      mask prompts: bus "CAN Bus"
      mask Display: disp(['Charge Port DC Voltage Sensor\n' bus]);
  Cooling Pump 1 : Subsystem  Commented=on  mask{nam='CoolPump1', bus='CAN1'}
      mask prompts: nam "Name"; bus "CAN Bus"
      mask init:
      | cb = gcb;
      | 
      | % --- Name Line
      | NameLine([cb '/CAN'], 'Inport', nam);
      mask Display: disp(['Water Pump: EMP WP29 (J1939)\n' nam '\n' bus]);
  Cooling Pump 2 : Subsystem  Commented=on  mask{nam='CoolPump2', bus='CAN1'}
      mask prompts: nam "Name"; bus "CAN Bus"
      mask init:
      | cb = gcb;
      | 
      | % --- Name Line
      | NameLine([cb '/CAN'], 'Inport', nam);
      mask Display: disp(['Water Pump: EMP WP29 (J1939)\n' nam '\n' bus]);
  EPAS : Subsystem  mask{nam='EPAS', bus='CAN1'}
      mask prompts: nam "Name"; bus "CAN Bus"
      mask init:
      | cb = gcb;
      | 
      | % --- Name Line
      | NameLine([cb '/CAN'], 'Inport', nam);
      mask Display: disp(['Display\n' nam '\n' bus]);
  Header : Blocks_lib/Header  width=Portrait  addtext=''
  Heater : Subsystem  Commented=on  mask{bus='CAN1'}
      mask prompts: bus "CAN Bus"
      mask Display: disp(['Heater: Mitsubishi EWH40Dx\n' bus]);
  Power Steering Pump Inverter : Subsystem  Commented=on  mask{nam='PSPInvtr', bus='CAN1'}
      mask prompts: nam "Name"; bus "CAN Bus"
      mask init:
      | cb = gcb;
      | 
      | % --- Name Line
      | NameLine([cb '/CAN'], 'Inport', nam);
      mask Display: disp(['Inverter: Sevcon HVLP-20\n' nam '\n' bus]);
  CAN : Outport  VectorParamsAs1DForOutWhenUnconnected=off
  wires:
  Bus Creator/1 -> CAN/1  "Other"
  Data/1 -> Power Steering Pump Inverter/1(Data), A/C Compressor/1(Data), Heater/1(Data), Cooling Pump 1/1(Data), Cooling Pump 2/1(Data), EPAS/1(Data), BCM1/1(Data), Charge Port DC Voltage Sensor/1(Data), BCM/1(Data)
  BCM/1(CAN) -> Bus Creator/1
  BCM1/1(CAN) -> Bus Creator/3
  Charge Port DC Voltage Sensor/1(CAN) -> Bus Creator/2
  EPAS/1(CAN) -> Bus Creator/4
